simulink model "workspace_270206023_23"  (R2023a)
settings: Solver=FixedStepDiscrete  StartTime=0.0  StopTime=inf  FixedStep=0.01  RelTol=1e-3
model workspace (MAT data in the model file):
  SEDAN = 1
  SUV = 0
  active = 1
  auto = 1
  close = 0
  cond_door_miss = 0
  cond_door_ok = 1
  fail_off = 0
  fail_on = 1
  ign_off = 0
  ign_on = 1
  key_off = 0
  key_on = 1
  manu = 0
  not_Active = 0
  open = 1
  recovery = 3
settings Model: Creator=Grachus  LastModifiedBy=Grachus

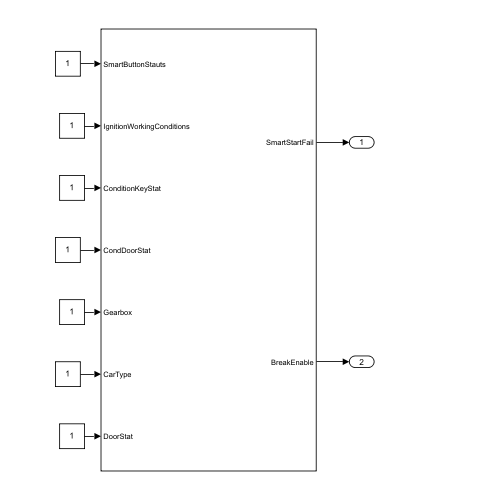
[thumbnail: Simulink's stored preview of the top-level diagram]
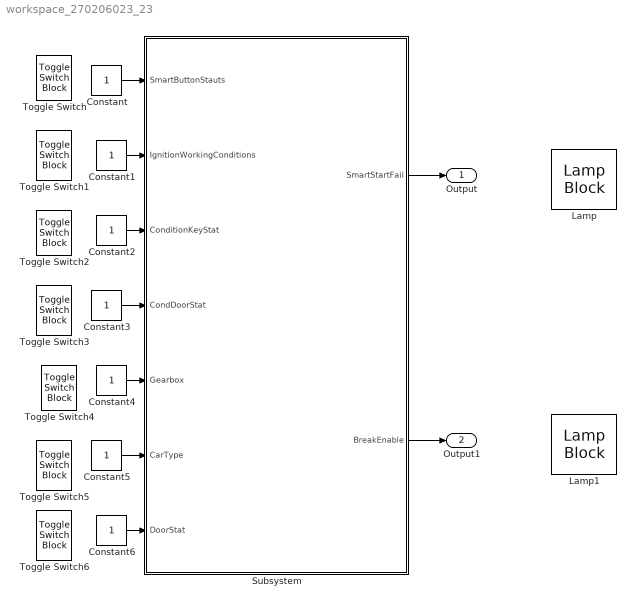
== system workspace_270206023_23 ==
  Constant{,1..6} (7 alike) : Constant
  Lamp : LampBlock  LabelPosition=Hide
  Lamp1 : LampBlock  LabelPosition=Hide
  Subsystem : Subsystem
  Toggle Switch{,1..6} (7 alike) : ToggleSwitchBlock
      settings: Values={{'Off', 'On'}, [0 1]}
  Output : Outport
  Output1 : Outport  Port=2
  wires:
  Constant/1 -> Subsystem/1(SmartButtonStauts)
  Constant1/1 -> Subsystem/2(IgnitionWorkingConditions)
  Constant2/1 -> Subsystem/3(ConditionKeyStat)
  Constant3/1 -> Subsystem/4(CondDoorStat)
  Constant4/1 -> Subsystem/5(Gearbox)
  Constant5/1 -> Subsystem/6(CarType)
  Constant6/1 -> Subsystem/7(DoorStat)
  Subsystem/1(SmartStartFail) -> Output/1
  Subsystem/2(BreakEnable) -> Output1/1

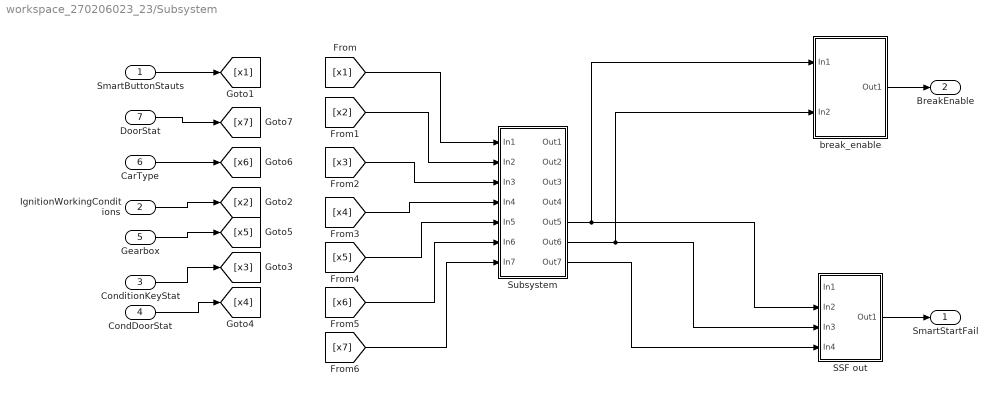
== system workspace_270206023_23/Subsystem ==
  SmartButtonStauts : Inport
  IgnitionWorkingConditions : Inport  Port=2
  ConditionKeyStat : Inport  Port=3
  CondDoorStat : Inport  Port=4
  Gearbox : Inport  Port=5
  CarType : Inport  Port=6
  DoorStat : Inport  Port=7
  SSF out : Subsystem
  Subsystem : Subsystem
  break_enable : Subsystem
  SmartStartFail : Outport
  BreakEnable : Outport  Port=2
  wires:
  SmartButtonStauts/1 -> [x1]
  IgnitionWorkingConditions/1 -> [x2]
  ConditionKeyStat/1 -> [x3]
  CondDoorStat/1 -> [x4]
  Gearbox/1 -> [x5]
  CarType/1 -> [x6]
  DoorStat/1 -> [x7]
  [x1] -> Subsystem/1(In1)
  [x2] -> Subsystem/2(In2)
  [x3] -> Subsystem/3(In3)
  [x4] -> Subsystem/4(In4)
  [x5] -> Subsystem/5(In5)
  [x6] -> Subsystem/6(In6)
  [x7] -> Subsystem/7(In7)
  Subsystem/5(Out5) -> break_enable/1(In1), SSF out/2(In2)
  Subsystem/6(Out6) -> break_enable/2(In2), SSF out/3(In3)
  Subsystem/7(Out7) -> SSF out/4(In4)
  SSF out/1(Out1) -> SmartStartFail/1
  break_enable/1(Out1) -> BreakEnable/1

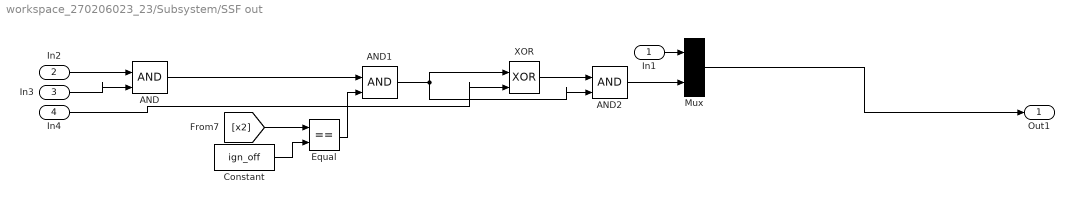
== system workspace_270206023_23/Subsystem/SSF out ==
  In1 : Inport
  In2 : Inport  Port=2
  In3 : Inport  Port=3
  In4 : Inport  Port=4
  AND : Logic  IconShape=distinctive  AllPortsSameDT=off  OutDataTypeStr=boolean
  AND1 : Logic  IconShape=distinctive  AllPortsSameDT=off  OutDataTypeStr=boolean
  AND2 : Logic  IconShape=distinctive  AllPortsSameDT=off  OutDataTypeStr=boolean
  Constant : Constant  Value=ign_off
  Equal : RelationalOperator  Operator===  OutDataTypeStr=boolean  RndMeth=Simplest  InputSameDT=off
  Mux : Mux  Inputs=2
  XOR : Logic  Operator=XOR  IconShape=distinctive  AllPortsSameDT=off  OutDataTypeStr=boolean
  Out1 : Outport
  wires:
  AND1/1 -> XOR/1, AND2/2
  AND2/1 -> Mux/2
  Equal/1 -> AND1/2
  XOR/1 -> AND2/1
  In2/1 -> AND/1
  Constant/1 -> Equal/2
  AND/1 -> AND1/1
  [x2] -> Equal/1
  In1/1 -> Mux/1
  In3/1 -> AND/2
  In4/1 -> XOR/2
  Mux/1 -> Out1/1

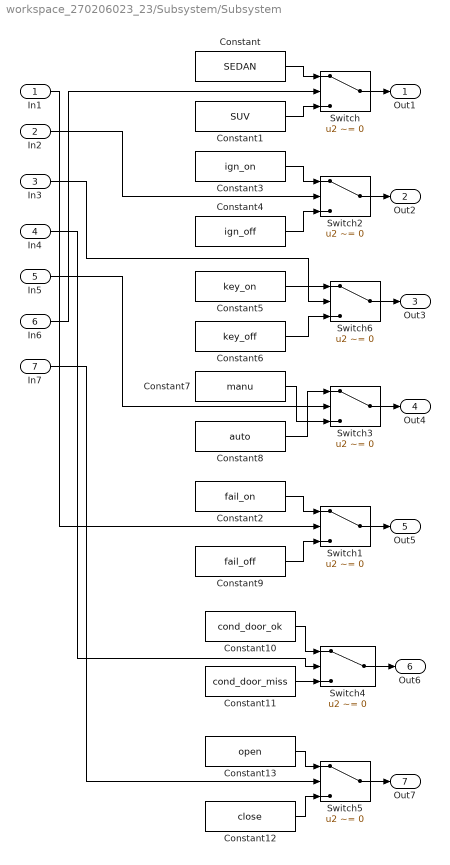
== system workspace_270206023_23/Subsystem/Subsystem ==
  In1 : Inport
  In2 : Inport  Port=2
  In3 : Inport  Port=3
  In4 : Inport  Port=4
  In5 : Inport  Port=5
  In6 : Inport  Port=6
  In7 : Inport  Port=7
  Constant : Constant  Value=SEDAN
  Constant1 : Constant  Value=SUV  SampleTime=-1
  Constant10 : Constant  Value=cond_door_ok  SampleTime=-1
  Constant11 : Constant  Value=cond_door_miss  SampleTime=-1
  Constant12 : Constant  Value=close  SampleTime=-1
  Constant13 : Constant  Value=open  SampleTime=-1
  Constant2 : Constant  Value=fail_on  SampleTime=-1
  Constant3 : Constant  Value=ign_on  SampleTime=-1
  Constant4 : Constant  Value=ign_off  SampleTime=-1
  Constant5 : Constant  Value=key_on  SampleTime=-1
  Constant6 : Constant  Value=key_off  SampleTime=-1
  Constant7 : Constant  Value=manu  SampleTime=-1
  Constant8 : Constant  Value=auto  SampleTime=-1
  Constant9 : Constant  Value=fail_off  SampleTime=-1
  Switch{,1..6} (7 alike) : Switch  Criteria=u2 ~= 0  SaturateOnIntegerOverflow=off  InputSameDT=off
  Out1 : Outport
  Out2 : Outport  Port=2
  Out3 : Outport  Port=3
  Out4 : Outport  Port=4
  Out5 : Outport  Port=5
  Out6 : Outport  Port=6
  Out7 : Outport  Port=7
  wires:
  Constant2/1 -> Switch1/1
  Constant/1 -> Switch/1
  Switch4/1 -> Out6/1
  Constant6/1 -> Switch6/3
  Switch6/1 -> Out3/1
  Switch5/1 -> Out7/1
  Switch1/1 -> Out5/1
  Constant8/1 -> Switch3/1
  Constant1/1 -> Switch/3
  In7/1 -> Switch5/2
  Constant9/1 -> Switch1/3
  Constant7/1 -> Switch3/3
  Constant3/1 -> Switch2/1
  Constant13/1 -> Switch5/1
  Constant4/1 -> Switch2/3
  Constant5/1 -> Switch6/1
  Constant12/1 -> Switch5/3
  Switch/1 -> Out1/1
  In4/1 -> Switch4/2
  Constant11/1 -> Switch4/3
  Constant10/1 -> Switch4/1
  Switch2/1 -> Out2/1
  In2/1 -> Switch2/2
  In6/1 -> Switch/2
  In5/1 -> Switch3/2
  In3/1 -> Switch6/2
  In1/1 -> Switch1/2
  Switch3/1 -> Out4/1

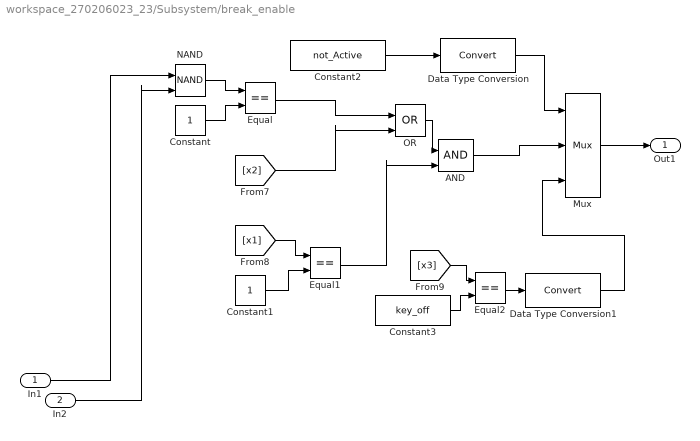
== system workspace_270206023_23/Subsystem/break_enable ==
  In1 : Inport
  In2 : Inport  Port=2
  AND : Logic  IconShape=distinctive  AllPortsSameDT=off  OutDataTypeStr=boolean
  Constant : Constant
  Constant1 : Constant
  Constant2 : Constant  Value=not_Active
  Constant3 : Constant  Value=key_off
  Data Type Conversion : DataTypeConversion  SaturateOnIntegerOverflow=off  RndMeth=Floor
  Data Type Conversion1 : DataTypeConversion  SaturateOnIntegerOverflow=off  RndMeth=Floor
  Equal : RelationalOperator  Operator===  OutDataTypeStr=boolean  RndMeth=Simplest  InputSameDT=off
  Equal1 : RelationalOperator  Operator===  OutDataTypeStr=boolean  RndMeth=Simplest  InputSameDT=off
  Equal2 : RelationalOperator  Operator===  OutDataTypeStr=boolean  RndMeth=Simplest  InputSameDT=off
  Mux : Mux  Inputs=3
  NAND : Logic  Operator=NAND  IconShape=distinctive  AllPortsSameDT=off  OutDataTypeStr=boolean
  OR : Logic  Operator=OR  IconShape=distinctive  AllPortsSameDT=off  OutDataTypeStr=boolean
  Out1 : Outport
  wires:
  Constant3/1 -> Equal2/2
  Constant1/1 -> Equal1/2
  [x3] -> Equal2/1
  [x1] -> Equal1/1
  Constant2/1 -> Data Type Conversion/1
  OR/1 -> AND/1
  [x2] -> OR/2
  Equal1/1 -> AND/2
  In1/1 -> NAND/1
  NAND/1 -> Equal/1
  AND/1 -> Mux/2
  Equal/1 -> OR/1
  Constant/1 -> Equal/2
  Mux/1 -> Out1/1
  In2/1 -> NAND/2
  Data Type Conversion/1 -> Mux/1
  Equal2/1 -> Data Type Conversion1/1
  Data Type Conversion1/1 -> Mux/3
